simulink model "simulink_slice"  (R2012b)
settings: Solver=ode45  StartTime=0.0  StopTime=10.0  RelTol=1e-3
libraries: xbsIndex_r4 x8, simulink x3
settings Model: Creator=paulp  LastModifiedBy=paulp

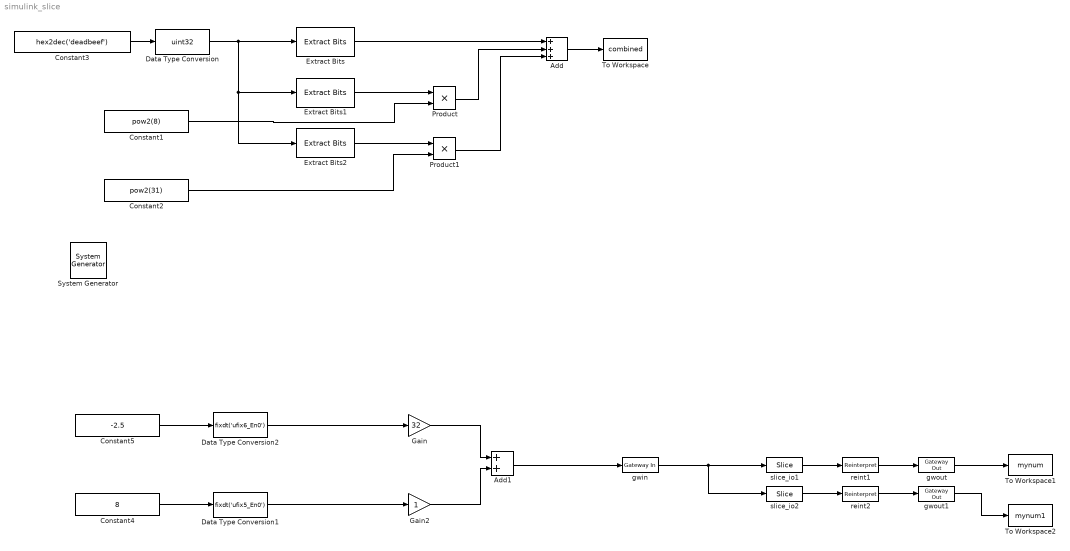
== system simulink_slice ==
  " System Generator" : xbsIndex_r4/ System Generator  Tag=genX  xilinxfamily=Kintex7  part=xc7k325t  speed=-3  package=fbg676  synthesis_tool=XST  clock_wrapper=Clock Enables  directory=./netlist  proj_type=Project Navigator  Synth_file=XST Defaults  Impl_file=ISE Defaults  testbench=off  simulink_period=1  sysclk_period=10  dcm_input_clock_period=10  incr_netlist=off  trim_vbits=Everywhere in SubSystem  dbl_ovrd=According to Block Masks  core_generation=According to Block Masks  run_coregen=off  deprecated_control=off  eval_field=0  block_type=sysgen
  Add : Sum  Inputs=+++  OutDataTypeStr=uint32
  Add1 : Sum  OutDataTypeStr=uint32
  Constant1 : Constant  Value=pow2(8)  OutDataTypeStr=uint32  LockScale=on
  Constant2 : Constant  Value=pow2(31)  OutDataTypeStr=uint32  LockScale=on
  Constant3 : Constant  Value=hex2dec('deadbeef')  OutDataTypeStr=uint32  LockScale=on
  Constant4 : Constant  Value=8  OutDataTypeStr=fixdt('ufix5_En0')  LockScale=on
  Constant5 : Constant  Value=-2.5  OutDataTypeStr=fixdt('sfix6_En3')  LockScale=on
  Data Type Conversion : DataTypeConversion  OutDataTypeStr=uint32
  Data Type Conversion1 : DataTypeConversion  OutDataTypeStr=fixdt('ufix5_En0')  LockScale=on
  Data Type Conversion2 : DataTypeConversion  OutDataTypeStr=fixdt('ufix6_En0')  LockScale=on
  Extract Bits : simulink/Logic and Bit Operations/Extract Bits  bitsToExtract=Range of bits  numBits=8  bitIdxRange=[0 3]  outScalingMode=Treat bit field as an integer
  Extract Bits1 : simulink/Logic and Bit Operations/Extract Bits  bitsToExtract=Range of bits  numBits=8  bitIdxRange=[8 30]  outScalingMode=Treat bit field as an integer
  Extract Bits2 : simulink/Logic and Bit Operations/Extract Bits  bitsToExtract=Range of bits  numBits=8  bitIdxRange=[31 31]  outScalingMode=Treat bit field as an integer
  Gain : Gain  Gain=32
  Gain2 : Gain
  Product : Product  RndMeth=Zero
  Product1 : Product  RndMeth=Zero
  To Workspace : ToWorkspace  VariableName=combined  SampleTime=-1  SaveFormat=Structure
  To Workspace1 : ToWorkspace  VariableName=mynum  SampleTime=-1  SaveFormat=Structure
  To Workspace2 : ToWorkspace  VariableName=mynum1  SampleTime=-1  SaveFormat=Structure
  gwin : xbsIndex_r4/Gateway In  gui_display_data_type=Fixed-point  arith_type=Unsigned  n_bits=32  bin_pt=0  preci_type=Single  exp_width=8  frac_width=24  quantization="Round  (unbiased: +/- Inf)"  overflow=Saturate  period=1  dbl_ovrd=off  timing_constraint=None  locs_specified=off  LOCs={}  UseAsADC=off  ADCChannel='1'  inherit_from_input=off  hdl_port=on  block_type=gatewayin
  gwout : xbsIndex_r4/Gateway Out  inherit_from_input=off  hdl_port=off  timing_constraint=None  locs_specified=off  LOCs={}  UseAsDAC=off  DACChannel='1'  block_type=gatewayout
  gwout1 : xbsIndex_r4/Gateway Out  inherit_from_input=off  hdl_port=off  timing_constraint=None  locs_specified=off  LOCs={}  UseAsDAC=off  DACChannel='1'  block_type=gatewayout
  reint1 : xbsIndex_r4/Reinterpret  force_arith_type=on  arith_type="Signed  (2's comp)"  force_bin_pt=on  bin_pt=3  block_type=reinterpret
  reint2 : xbsIndex_r4/Reinterpret  force_arith_type=on  arith_type=Unsigned  force_bin_pt=on  bin_pt=0  block_type=reinterpret
  slice_io1 : xbsIndex_r4/Slice  nbits=6  boolean_output=off  mode=Lower Bit Location + Width  bit1=0  base1=MSB of Input  bit0=5  base0=LSB of Input  dbl_ovrd=off  block_type=slice
  slice_io2 : xbsIndex_r4/Slice  nbits=5  boolean_output=off  mode=Lower Bit Location + Width  bit1=0  base1=MSB of Input  bit0=0  base0=LSB of Input  dbl_ovrd=off  block_type=slice
  wires:
  Constant3/1 -> Data Type Conversion/1
  Extract Bits1/1 -> Product/1
  Extract Bits2/1 -> Product1/1
  Constant1/1 -> Product/2
  Constant2/1 -> Product1/2
  Product1/1 -> Add/3
  Product/1 -> Add/2
  Extract Bits/1 -> Add/1
  Add/1 -> To Workspace/1
  Data Type Conversion/1 -> Extract Bits1/1, Extract Bits2/1, Extract Bits/1
  Constant4/1 -> Data Type Conversion1/1
  Constant5/1 -> Data Type Conversion2/1
  Data Type Conversion1/1 -> Gain2/1
  Data Type Conversion2/1 -> Gain/1
  Gain/1 -> Add1/1
  Gain2/1 -> Add1/2
  gwin/1 -> slice_io2/1, slice_io1/1
  Add1/1 -> gwin/1
  slice_io1/1 -> reint1/1
  slice_io2/1 -> reint2/1
  reint1/1 -> gwout/1
  gwout/1 -> To Workspace1/1
  reint2/1 -> gwout1/1
  gwout1/1 -> To Workspace2/1
